simulink model "Citation"  (Simulink 10.1)
settings: Solver=ode5  StartTime=0.0  StopTime=inf  FixedStep=0.01  RelTol=1e-3  EnableMultiTasking=on
values from neighbouring files (symbols this model uses):
  S = 12.9900    (= 12.99)    [FTFC.m]
  Vw915 = 0    [initcit.m]
  winddir = 45*(pi/180)    (= 0.785398163397)    [initcit.m]
  x0 = []    [cessnac550_3d_sfnc.m]    (also in sfunxyz.m)
undefined symbols (not defined in the file or in its folder): chord, cv1, cv2, cv3, cv4, deltagmax1, deltagmax2, deltagmax3, deltagmax4, Deng, ealphag, ealphas, g0, hDME, hGS, kt1, kt2, kt3, lh, massinit, matbuaf, matdaf, matdam, matdbbf, matdeaf, matdgaf, matdqaf, matduaf, matdwaw, matedhr, mateif, matelhr, matemhr, matemv1, matemv2, matemve, matetam, mateuaf, matfaaf, matfaxl, matff, matibaf, matibmh, matipaf, matipmh, matiraf, matiuaf, matiwaf, matlaf, matlam, matleaf, matleam, matlgaf, matlqaf, matluaf, matmaaf, matmaam, matmaf, matmam, matmbbf ... (+74)
undefined symbols (not defined in the file): matibb
libraries: simulink x12, vrlib x1
(part 4 of 5)

== system Citation/Cessna Citation 500/Citation model DASMAT/AIRCRAFT MODEL/LANDING GEAR/Landing Gear model/Right Main Gear/Axes Transformation Heading attached vertical axis to body axis ==
  Fmu FS FV phi theta : Inport
  FX : Fcn  Expr=-cos(u[5])*u[1]+0*u[2]+sin(u[5])*u[3]
  FY : Fcn  Expr=-sin(u[5])*sin(u[4])*u[1]-cos(u[4])*u[2]-cos(u[5])*sin(u[4])*u[3]
  FZ : Fcn  Expr=-sin(u[5])*cos(u[4])*u[1]+sin(u[4])*u[2]-cos(u[5])*cos(u[4])*u[3]
  Mux1 : Mux  Inputs=3
  FX FY FZ : Outport
  wires:
  Fmu FS FV phi theta/1 -> FX/1, FY/1, FZ/1
  FX/1 -> Mux1/1
  FY/1 -> Mux1/2
  FZ/1 -> Mux1/3
  Mux1/1 -> FX FY FZ/1

== system Citation/Cessna Citation 500/Citation model DASMAT/AIRCRAFT MODEL/LANDING GEAR/Landing Gear model/Right Main Gear/Calculation of the Moments ==
  FX FY FZ : Inport
  L : Fcn  Expr=0*u[1]-zl2*u[2]+yl2*u[3]
  M : Fcn  Expr=zl2*u[1]+0*u[2]-xl2*u[3]
  Mux2 : Mux  Inputs=3
  N : Fcn  Expr=-yl2*u[1]+xl2*u[2]+0*u[3]
  L M N : Outport
  wires:
  L/1 -> Mux2/1
  M/1 -> Mux2/2
  N/1 -> Mux2/3
  FX FY FZ/1 -> M/1, L/1, N/1
  Mux2/1 -> L M N/1

== system Citation/Cessna Citation 500/Citation model DASMAT/AIRCRAFT MODEL/LANDING GEAR/Landing Gear model/Right Main Gear/FV Vertical Force ==
  In1 : Inport
  B : Fcn  Expr=(u[2]/kt2)-u[1]-deltagmax2
  C : Fcn  Expr=(deltagmax2/kt2)*(P2+u[2]-(kt2*u[1]))
  FD damping force : Fcn  Expr=cv2*u[1]
  FV : Fcn  Expr=kt2*(u[1]-u[2])
  FV No ground contact : Constant  Value=0
  Mux1 : Mux  Inputs=2
  Mux2 : Mux  Inputs=2
  Mux3 : Mux  Inputs=2
  No negative  Strut deflection : Saturate  UpperLimit=inf  LowerLimit=0
  Prevent Earth  from pulling a/c when FD>FV : Saturate  UpperLimit=inf  LowerLimit=0
  Strut deflection : Fcn  Expr=0.5*(-u[1]-sqrt(u[1]*u[1]+4*u[2]))
  Switch1 : Switch  SaturateOnIntegerOverflow=on  InputSameDT=on
  deltag : Fcn  Expr=zl2-u[10]-xl2*sin(u[8])+yl2*sin(u[7])
  deltagdot : Fcn  Expr=-u[13]-xl2*u[2]*cos(u[8])+yl2*u[1]*cos(u[7])
  Out1 : Outport
  wires:
  In1/1 -> deltag/1, deltagdot/1
  deltagdot/1 -> FD damping force/1
  Strut deflection/1 -> No negative  Strut deflection/1
  FD damping force/1 -> Mux1/2
  Mux1/1 -> B/1, C/1
  B/1 -> Mux2/1
  C/1 -> Mux2/2
  Mux2/1 -> Strut deflection/1
  Mux3/1 -> FV/1
  No negative  Strut deflection/1 -> Mux3/2
  deltag/1 -> Mux1/1, Mux3/1, Switch1/2
  FV/1 -> Prevent Earth  from pulling a/c when FD>FV/1
  FV No ground contact/1 -> Switch1/3
  Prevent Earth  from pulling a/c when FD>FV/1 -> Switch1/1
  Switch1/1 -> Out1/1

== system Citation/Cessna Citation 500/Citation model DASMAT/AIRCRAFT MODEL/LANDING GEAR/Landing Gear model/Tail Scraper/Axes Transformation Heading attached vertical axis to body axis ==
  Fmu FS FV phi theta : Inport
  FX : Fcn  Expr=-cos(u[5])*u[1]+0*u[2]+sin(u[5])*u[3]
  FY : Fcn  Expr=-sin(u[5])*sin(u[4])*u[1]-cos(u[4])*u[2]-cos(u[5])*sin(u[4])*u[3]
  FZ : Fcn  Expr=-sin(u[5])*cos(u[4])*u[1]+sin(u[4])*u[2]-cos(u[5])*cos(u[4])*u[3]
  Mux1 : Mux  Inputs=3
  FX FY FZ : Outport
  wires:
  Fmu FS FV phi theta/1 -> FX/1, FY/1, FZ/1
  FX/1 -> Mux1/1
  FY/1 -> Mux1/2
  FZ/1 -> Mux1/3
  Mux1/1 -> FX FY FZ/1

== system Citation/Cessna Citation 500/Citation model DASMAT/AIRCRAFT MODEL/LANDING GEAR/Landing Gear model/Tail Scraper/Calculation of the Moments ==
  FX FY FZ : Inport
  L : Fcn  Expr=0*u[1]-zl4*u[2]+yl4*u[3]
  M : Fcn  Expr=zl4*u[1]+0*u[2]-xl4*u[3]
  Mux2 : Mux  Inputs=3
  N : Fcn  Expr=-yl4*u[1]+xl4*u[2]+0*u[3]
  L M N : Outport
  wires:
  L/1 -> Mux2/1
  M/1 -> Mux2/2
  N/1 -> Mux2/3
  FX FY FZ/1 -> M/1, L/1, N/1
  Mux2/1 -> L M N/1

== system Citation/Cessna Citation 500/Citation model DASMAT/AIRCRAFT MODEL/LANDING GEAR/Landing Gear model/Tail Scraper/FV Vertical Force ==
  In1 : Inport
  FD damping force : Fcn  Expr=cv4*u[1]
  FV : Fcn  Expr=P4*u[1]+u[2]
  FV No ground contact : Constant  Value=0
  Max Strut Deflection : Saturate  UpperLimit=deltagmax4  LowerLimit=-inf
  Mux1 : Mux  Inputs=2
  Prevent Earth  from pulling a/c when FD>FV : Saturate  UpperLimit=inf  LowerLimit=0
  Scope6 : Scope
  Switch : Switch  SaturateOnIntegerOverflow=on  InputSameDT=on
  deltag : Fcn  Expr=zl4-u[10]-xl4*sin(u[8])+yl4*sin(u[7])
  deltagdot : Fcn  Expr=-u[13]-xl4*u[2]*cos(u[8])+yl4*u[1]*cos(u[7])
  Out1 : Outport
  wires:
  In1/1 -> deltag/1, deltagdot/1
  deltagdot/1 -> FD damping force/1
  deltag/1 -> Max Strut Deflection/1
  Max Strut Deflection/1 -> Scope6/1, Mux1/1, Switch/2
  Mux1/1 -> FV/1
  FD damping force/1 -> Mux1/2
  FV/1 -> Prevent Earth  from pulling a/c when FD>FV/1
  Prevent Earth  from pulling a/c when FD>FV/1 -> Switch/1
  FV No ground contact/1 -> Switch/3
  Switch/1 -> Out1/1

== system Citation/Cessna Citation 500/Citation model DASMAT/AIRCRAFT MODEL/WIND/TURBULENCE/Logarithmic Wind model/Logarithmic Wind model/Vwind915 ==
  Constant : Constant  Value=0
  Parameter : Integrator  InitialCondition=Vw915
  Out1 : Outport
  wires:
  Constant/1 -> Parameter/1
  Parameter/1 -> Out1/1

== system Citation/Cessna Citation 500/Citation model DASMAT/AIRCRAFT MODEL/WIND/TURBULENCE/Logarithmic Wind model/Logarithmic Wind model/Windddirection ==
  Constant : Constant  Value=0
  Parameter : Integrator  InitialCondition=winddir
  Out1 : Outport
  wires:
  Constant/1 -> Parameter/1
  Parameter/1 -> Out1/1

== system Citation/Cessna Citation 500/Citation model DASMAT/AIRCRAFT MODEL/AFM/Aeromod/SubSystem/model/CDCAL ==
  in_1 : Inport
  Abs : Abs  SaturateOnIntegerOverflow=on
  Abs1 : Abs  SaturateOnIntegerOverflow=on
  CD : Sum  Inputs=++++++++  InputSameDT=on  SaturateOnIntegerOverflow=on  OutDataTypeStr=Inherit: Same as first input
  CDAF : Lookup2D  RowIndex=matdaf(2:23,1)  ColumnIndex=matdaf(1,2:23)  Table=matdaf(2:23,2:23)  SaturateOnIntegerOverflow=on  InputSameDT=on
  CDAM : Lookup2D  RowIndex=matdam(2:23,1)  ColumnIndex=matdam(1,2:23)  Table=matdam(2:23,2:23)  SaturateOnIntegerOverflow=on  InputSameDT=on
  CDBAS : Sum  InputSameDT=on  SaturateOnIntegerOverflow=on  OutDataTypeStr=Inherit: Same as first input
  CDBBF : Lookup2D  RowIndex=matdbbf(2:18,1)  ColumnIndex=matdbbf(1,2:18)  Table=matdbbf(2:18,2:18)  SaturateOnIntegerOverflow=on  InputSameDT=on
  CDDE : Product  InputSameDT=on  SaturateOnIntegerOverflow=on  OutDataTypeStr=Inherit: Same as first input
  CDEAF : Lookup2D  RowIndex=matdeaf(2:23,1)  ColumnIndex=matdeaf(1,2:23)  Table=matdeaf(2:23,2:23)  SaturateOnIntegerOverflow=on  InputSameDT=on
  CDGAF : Lookup2D  RowIndex=matdgaf(2:4,1)  ColumnIndex=matdgaf(1,2:4)  Table=matdgaf(2:4,2:4)  SaturateOnIntegerOverflow=on  InputSameDT=on
  CDGE : Product  InputSameDT=on  SaturateOnIntegerOverflow=on  OutDataTypeStr=Inherit: Same as first input
  CDQ : Product  InputSameDT=on  SaturateOnIntegerOverflow=on  OutDataTypeStr=Inherit: Same as first input
  CDQAF : Lookup2D  RowIndex=matdqaf(2:23,1)  ColumnIndex=matdqaf(1,2:23)  Table=matdqaf(2:23,2:23)  SaturateOnIntegerOverflow=on  InputSameDT=on
  CDR : Product  Inputs=3  InputSameDT=on  SaturateOnIntegerOverflow=on  OutDataTypeStr=Inherit: Same as first input
  CDRUAF : Lookup2D  RowIndex=matruaf(2:3,1)  ColumnIndex=matruaf(1,2:3)  Table=matruaf(2:3,2:3)  SaturateOnIntegerOverflow=on  InputSameDT=on
  CDUAF : Lookup2D  RowIndex=matduaf(2:23,1)  ColumnIndex=matduaf(1,2:23)  Table=matduaf(2:23,2:23)  SaturateOnIntegerOverflow=on  InputSameDT=on
  CDUC : Product  InputSameDT=on  SaturateOnIntegerOverflow=on  OutDataTypeStr=Inherit: Same as first input
  CDWAW : Lookup2D  RowIndex=matdwaw(2:7,1)  ColumnIndex=matdwaw(1,2:7)  Table=matdwaw(2:7,2:7)  SaturateOnIntegerOverflow=on  InputSameDT=on
  Demux : Demux  Outputs=[1 1 1 1 1 1 1 1 1 1 1 1 1 1 1 1 1 1]
      settings: DisplayOption=none
  KBASD : Subsystem
  KGEDHR : Lookup  InputValues=matedhr(1,:)  Table=matedhr(2,:)  SaturateOnIntegerOverflow=on
  KUUT : Lookup  InputValues=matuut(1,:)  Table=matuut(2,:)  SaturateOnIntegerOverflow=on
  Prod : Product  InputSameDT=on  SaturateOnIntegerOverflow=on  OutDataTypeStr=Inherit: Same as first input
  Terminator_{1..7} (7 alike) : Terminator
  out_1 : Outport
  wires:
  Demux/16 -> Terminator_7/1
  Demux/13 -> Terminator_6/1
  Demux/12 -> Terminator_5/1
  Demux/11 -> Terminator_4/1
  Demux/6 -> Terminator_3/1
  Demux/3 -> Terminator_2/1
  Demux/1 -> Terminator_1/1
  Demux/7 -> KBASD/1(hcg), KGEDHR/1
  Demux/18 -> KBASD/3(VEAS)
  Demux/2 -> CDQ/1
  Demux/5 -> Abs1/1
  Demux/8 -> CDDE/1
  Demux/9 -> Abs/1
  Demux/15 -> KUUT/1
  Demux/17 -> CDAM/1
  KUUT/1 -> CDUC/2
  CDGAF/1 -> CDGE/1
  CDR/1 -> CD/6
  CDQ/1 -> CD/5
  CDWAW/1 -> CD/3
  CDDE/1 -> CD/2
  CDRUAF/1 -> CDR/3
  CDQAF/1 -> CDQ/2
  CDEAF/1 -> CDDE/2
  Abs/1 -> CDWAW/1
  Abs1/1 -> CDBBF/2
  CD/1 -> out_1/1
  Demux/10 -> CDR/1, CDR/2
  Demux/14 -> CDAF/1, CDRUAF/1, CDUAF/1, CDGAF/1, CDQAF/1, CDBBF/1, CDEAF/1, KBASD/2(deltaf)
  KGEDHR/1 -> CDGE/2
  Demux/4 -> CDRUAF/2, CDUAF/2, CDGAF/2, CDQAF/2, CDWAW/2, CDEAF/2, CDAF/2, CDAM/2
  CDAF/1 -> Prod/1
  KBASD/1(KBASD) -> Prod/2
  CDUAF/1 -> CDUC/1
  CDUC/1 -> CD/7
  CDGE/1 -> CD/8
  CDBBF/1 -> CD/4
  Prod/1 -> CDBAS/2
  CDAM/1 -> CDBAS/1
  CDBAS/1 -> CD/1
  in_1/1 -> Demux/1

== system Citation/Cessna Citation 500/Citation model DASMAT/AIRCRAFT MODEL/AFM/Aeromod/SubSystem/model/CLCAL ==
  in_1 : Inport
  CL : Sum  Inputs=+++++  InputSameDT=on  SaturateOnIntegerOverflow=on  OutDataTypeStr=Inherit: Same as first input
  CLADOT : Product  InputSameDT=on  SaturateOnIntegerOverflow=on  OutDataTypeStr=Inherit: Same as first input
  CLAF : Lookup2D  RowIndex=matlaf(2:23,1)  ColumnIndex=matlaf(1,2:23)  Table=matlaf(2:23,2:23)  SaturateOnIntegerOverflow=on  InputSameDT=on
  CLAM : Lookup2D  RowIndex=matlam(2:23,1)  ColumnIndex=matlam(1,2:23)  Table=matlam(2:23,2:23)  SaturateOnIntegerOverflow=on  InputSameDT=on
  CLBAS : Sum  InputSameDT=on  SaturateOnIntegerOverflow=on  OutDataTypeStr=Inherit: Same as first input
  CLDE : Product  InputSameDT=on  SaturateOnIntegerOverflow=on  OutDataTypeStr=Inherit: Same as first input
  CLEAF : Lookup2D  RowIndex=matleaf(2:23,1)  ColumnIndex=matleaf(1,2:23)  Table=matleaf(2:23,2:23)  SaturateOnIntegerOverflow=on  InputSameDT=on
  CLEAM : Lookup2D  RowIndex=matleam(2:3,1)  ColumnIndex=matleam(1,2:3)  Table=matleam(2:3,2:3)  SaturateOnIntegerOverflow=on  InputSameDT=on
  CLFAAF : Lookup2D  RowIndex=matfaaf(2:23,1)  ColumnIndex=matfaaf(1,2:23)  Table=matfaaf(2:23,2:23)  SaturateOnIntegerOverflow=on  InputSameDT=on
  CLGAF : Lookup2D  RowIndex=matlgaf(2:4,1)  ColumnIndex=matlgaf(1,2:4)  Table=matlgaf(2:4,2:4)  SaturateOnIntegerOverflow=on  InputSameDT=on
  CLGE : Product  InputSameDT=on  SaturateOnIntegerOverflow=on  OutDataTypeStr=Inherit: Same as first input
  CLGEAF : Subsystem
  CLQ : Product  Inputs=3  InputSameDT=on  SaturateOnIntegerOverflow=on  OutDataTypeStr=Inherit: Same as first input
  CLQAF : Lookup2D  RowIndex=matlqaf(2:23,1)  ColumnIndex=matlqaf(1,2:23)  Table=matlqaf(2:23,2:23)  SaturateOnIntegerOverflow=on  InputSameDT=on
  CLQUAF : Lookup2D  RowIndex=matqlaf(2:3,1)  ColumnIndex=matqlaf(1,2:3)  Table=matqlaf(2:3,2:3)  SaturateOnIntegerOverflow=on  InputSameDT=on
  CLUAF : Lookup2D  RowIndex=matluaf(2:23,1)  ColumnIndex=matluaf(1,2:23)  Table=matluaf(2:23,2:23)  SaturateOnIntegerOverflow=on  InputSameDT=on
  CLUC : Product  InputSameDT=on  SaturateOnIntegerOverflow=on  OutDataTypeStr=Inherit: Same as first input
  Demux : Demux  Outputs=[1 1 1 1 1 1 1 1 1 1 1 1 1 1 1 1 1 1]
      settings: DisplayOption=none
  Gain : Gain  Gain=0.01  SaturateOnIntegerOverflow=on  OutDataTypeStr=Inherit: Same as input  ParamDataTypeStr=Inherit: Same as input
  KFAXL : Lookup  InputValues=matfaxl(1,:)  Table=matfaxl(2,:)  SaturateOnIntegerOverflow=on
  KGELHR : Lookup  InputValues=matelhr(1,:)  Table=matelhr(2,:)  SaturateOnIntegerOverflow=on
  KQXL : Lookup  InputValues=matqxl(1,:)  Table=matqxl(2,:)  SaturateOnIntegerOverflow=on
  KUUT : Lookup  InputValues=matuut(1,:)  Table=matuut(2,:)  SaturateOnIntegerOverflow=on
  Prod : Product  InputSameDT=on  SaturateOnIntegerOverflow=on  OutDataTypeStr=Inherit: Same as first input
  SP0 : Subsystem
  Sum : Sum  InputSameDT=on  SaturateOnIntegerOverflow=on  OutDataTypeStr=Inherit: Same as first input
  Sum1 : Sum  Inputs=2  InputSameDT=on  SaturateOnIntegerOverflow=on  OutDataTypeStr=Inherit: Same as first input
  Sum2 : Sum  Inputs=2  InputSameDT=on  SaturateOnIntegerOverflow=on  OutDataTypeStr=Inherit: Same as first input
  Terminator_{1..10} (10 alike) : Terminator
  out_1 : Outport
  out_2 : Outport  Port=2
  wires:
  Demux/18 -> Terminator_10/1
  Demux/13 -> Terminator_9/1
  Demux/12 -> Terminator_8/1
  Demux/11 -> Terminator_7/1
  Demux/10 -> Terminator_6/1
  Demux/9 -> Terminator_5/1
  Demux/6 -> Terminator_4/1
  Demux/5 -> Terminator_3/1
  Demux/3 -> Terminator_2/1
  Demux/1 -> Terminator_1/1
  CLADOT/1 -> out_2/1
  CLFAAF/1 -> CLADOT/1
  CLAF/1 -> CLBAS/2
  CLDE/1 -> CL/2
  Sum/1 -> CLDE/1
  SP0/1(SP0) -> CLDE/2
  CLQ/1 -> CL/3
  CL/1 -> out_1/1
  CLQUAF/1 -> Prod/2
  Sum1/1 -> CLUC/1
  CLQAF/1 -> CLQ/2
  Prod/1 -> Sum1/2
  CLUAF/1 -> Sum1/1
  CLGAF/1 -> Sum2/1
  KGELHR/1 -> CLGE/2
  KFAXL/1 -> Gain/1
  Gain/1 -> CLADOT/2
  Demux/14 -> CLAF/1, CLEAF/1, CLQAF/1, CLUAF/1, CLQUAF/1, CLGAF/1, CLGEAF/2(deltaf), CLFAAF/1
  CLEAF/1 -> Sum/2
  CLEAM/1 -> Sum/1
  CLUC/1 -> CL/4
  CLGE/1 -> CL/5
  CLGEAF/1(CLGEAF) -> Sum2/2
  in_1/1 -> Demux/1
  Demux/17 -> CLAM/1, CLEAM/1
  Demux/4 -> CLAM/2, CLAF/2, CLEAM/2, CLEAF/2, CLQAF/2, CLUAF/2, CLQUAF/2, CLGAF/2, CLGEAF/1(alpha), CLFAAF/2
  CLBAS/1 -> CL/1
  Demux/2 -> CLQ/1, Prod/1
  KQXL/1 -> CLQ/3
  KUUT/1 -> CLUC/2
  CLAM/1 -> CLBAS/1
  Demux/15 -> KQXL/1, KUUT/1
  Sum2/1 -> CLGE/1
  Demux/16 -> KFAXL/1
  Demux/8 -> SP0/1(deltae)
  Demux/7 -> KGELHR/1

== system Citation/Cessna Citation 500/Citation model DASMAT/AIRCRAFT MODEL/AFM/Aeromod/SubSystem/model/CLLCAL ==
  in_1 : Inport
  Abs : Abs  SaturateOnIntegerOverflow=on
  CIBAB : Subsystem  mask(3-D Table Lookup){xindex=matibb(2:5,1), yindex=matibb(1,2:4), zindex=matibb(1,5:7), table=matibb(2:5,2:10)}
      mask prompts: xindex "X Index"; yindex "Y Index"; zindex "Z Index"
      mask help:
      | Three Dimensional Table Lookup
      | The first, second and third input corresponds to the X,Y and Z Index
      mask Help: This block returns a linearly interpolated intersection from the table using the X index (which corresponds to the rows of the table), the Y index (which corresponds to the columns of the table) and the Z index.  Extrapolation is used.
      mask Display: plot(-10,-10,110,110,[90,50,10],[90,40,30],[90,50,10],[50,26,20],[90,50,10],[22,13,10])
  CIBAF : Lookup2D  RowIndex=matibaf(2:4,1)  ColumnIndex=matibaf(1,2:4)  Table=matibaf(2:4,2:4)  SaturateOnIntegerOverflow=on  InputSameDT=on
  CIBMH : Lookup2D  RowIndex=matibmh(2:10,1)  ColumnIndex=matibmh(1,2:10)  Table=matibmh(2:10,2:10)  SaturateOnIntegerOverflow=on  InputSameDT=on
  CIPAF : Lookup2D  RowIndex=matipaf(2:3,1)  ColumnIndex=matipaf(1,2:3)  Table=matipaf(2:3,2:3)  SaturateOnIntegerOverflow=on  InputSameDT=on
  CIPMH : Lookup2D  RowIndex=matipmh(2:10,1)  ColumnIndex=matipmh(1,2:10)  Table=matipmh(2:10,2:10)  SaturateOnIntegerOverflow=on  InputSameDT=on
  CIRAF : Lookup2D  RowIndex=matiraf(2:4,1)  ColumnIndex=matiraf(1,2:4)  Table=matiraf(2:4,2:4)  SaturateOnIntegerOverflow=on  InputSameDT=on
  CIRUAF : Lookup2D  RowIndex=matiuaf(2:3,1)  ColumnIndex=matiuaf(1,2:3)  Table=matiuaf(2:3,2:3)  SaturateOnIntegerOverflow=on  InputSameDT=on
  CIRUMH : Lookup2D  RowIndex=matrumh(2:10,1)  ColumnIndex=matrumh(1,2:10)  Table=matrumh(2:10,2:10)  SaturateOnIntegerOverflow=on  InputSameDT=on
  CIWAF : Lookup2D  RowIndex=matiwaf(2:3,1)  ColumnIndex=matiwaf(1,2:3)  Table=matiwaf(2:3,2:3)  SaturateOnIntegerOverflow=on  InputSameDT=on
  CIWTAM : Lookup2D  RowIndex=matwtam(2:3,1)  ColumnIndex=matwtam(1,2:3)  Table=matwtam(2:3,2:3)  SaturateOnIntegerOverflow=on  InputSameDT=on
  CLL : Sum  Inputs=+++++++  InputSameDT=on  SaturateOnIntegerOverflow=on  OutDataTypeStr=Inherit: Same as first input
  CLLB : Product  InputSameDT=on  SaturateOnIntegerOverflow=on  OutDataTypeStr=Inherit: Same as first input
  CLLDA : Product  InputSameDT=on  SaturateOnIntegerOverflow=on  OutDataTypeStr=Inherit: Same as first input
  CLLDR : Product  InputSameDT=on  SaturateOnIntegerOverflow=on  OutDataTypeStr=Inherit: Same as first input
  CLLGE : Product  Inputs=3  InputSameDT=on  SaturateOnIntegerOverflow=on  OutDataTypeStr=Inherit: Same as first input
  CLLGUST : Mux  Inputs=8
  CLLP : Product  InputSameDT=on  SaturateOnIntegerOverflow=on  OutDataTypeStr=Inherit: Same as first input
  CLLR : Product  InputSameDT=on  SaturateOnIntegerOverflow=on  OutDataTypeStr=Inherit: Same as first input
  CLLTRIM : Product  InputSameDT=on  SaturateOnIntegerOverflow=on  OutDataTypeStr=Inherit: Same as first input
  Demux1 : Demux  Outputs=[1 1 1 1 1 1 1 1 1 1 1 1 1 1 1 1 1 1]
      settings: DisplayOption=none
  LFACT : Subsystem
  LROLL : Lookup  InputValues=mateif(1,:)  Table=mateif(2,:)  SaturateOnIntegerOverflow=on
  Sum : Sum  Inputs=+++  InputSameDT=on  SaturateOnIntegerOverflow=on  OutDataTypeStr=Inherit: Same as first input
  Sum1 : Sum  InputSameDT=on  SaturateOnIntegerOverflow=on  OutDataTypeStr=Inherit: Same as first input
  Sum2 : Sum  InputSameDT=on  SaturateOnIntegerOverflow=on  OutDataTypeStr=Inherit: Same as first input
  Terminator_{1..7} (7 alike) : Terminator
  "neg " : Gain  Gain=-1  SaturateOnIntegerOverflow=on  OutDataTypeStr=Inherit: Same as input  ParamDataTypeStr=Inherit: Same as input
  zero : Constant  Value=0
  out_1 : Outport
  out_2 : Outport  Port=2
  wires:
  Demux1/18 -> Terminator_7/1
  Demux1/16 -> Terminator_6/1
  Demux1/15 -> Terminator_5/1
  Demux1/13 -> Terminator_4/1
  Demux1/11 -> Terminator_3/1
  Demux1/8 -> Terminator_2/1
  Demux1/2 -> Terminator_1/1
  Sum/1 -> CLLGUST/3, CLLB/2
  LFACT/1(LFACT) -> CLLGE/3
  LROLL/1 -> CLLGE/2
  CLL/1 -> out_1/1
  CLLB/1 -> CLL/1
  CIWTAM/1 -> CLLTRIM/2
  CIWAF/1 -> CLLDA/2
  Sum1/1 -> CLLDR/2
  CIRUMH/1 -> Sum1/2
  Abs/1 -> CIBAB/1(x0)
  CIRUAF/1 -> Sum1/1
  CIBAF/1 -> Sum/1
  CIPAF/1 -> Sum2/1
  CIPMH/1 -> Sum2/2
  Demux1/14 -> CIBAF/1, CIRUAF/1, CIRAF/1, LROLL/1, CIPAF/1, CIWAF/1, CIBAB/3(z0)
  Demux1/5 -> CLLB/1, Abs/1, CLLGE/1
  Demux1/4 -> CIWAF/2, CIRUAF/2, CIPAF/2, CIRAF/2, CIWTAM/2, CIBAB/2(y0), CIBAF/2
  zero/1 -> CLLGUST/2, CLLGUST/5, CLLGUST/6, CLLGUST/4, CLLGUST/1
  CLLGUST/1 -> out_2/1
  CIRAF/1 -> "neg "/1, CLLR/2
  Sum2/1 -> CLLGUST/8, CLLP/2
  "neg "/1 -> CLLGUST/7
  in_1/1 -> Demux1/1
  CLLGE/1 -> CLL/7
  CLLR/1 -> CLL/6
  CLLTRIM/1 -> CLL/4
  CLLDA/1 -> CLL/2
  Demux1/12 -> CLLTRIM/1
  Demux1/10 -> CLLDR/1
  Demux1/9 -> CLLDA/1
  Demux1/1 -> CLLP/1
  Demux1/3 -> CLLR/1
  CIBMH/1 -> Sum/2
  CIBAB/1(out_1) -> Sum/3
  Demux1/17 -> CIRUMH/2, CIWTAM/1, CIPMH/2, CIBMH/2
  Demux1/6 -> CIRUMH/1, CIPMH/1, CIBMH/1
  Demux1/7 -> LFACT/1(hcg)
  CLLP/1 -> CLL/5
  CLLDR/1 -> CLL/3

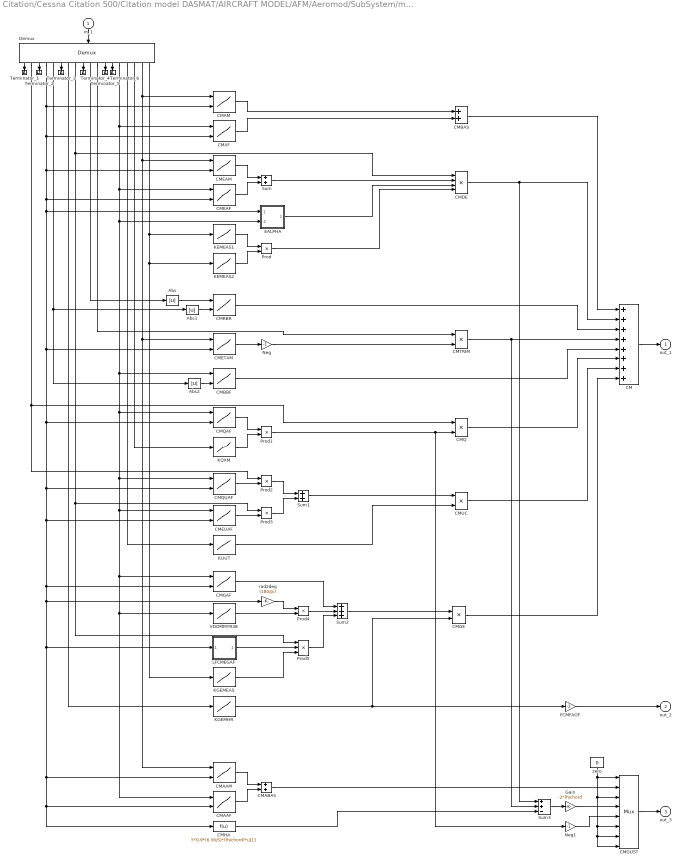
== system Citation/Cessna Citation 500/Citation model DASMAT/AIRCRAFT MODEL/AFM/Aeromod/SubSystem/model/CMCAL ==
  in_1 : Inport
  Abs : Abs  SaturateOnIntegerOverflow=on
  Abs1 : Abs  SaturateOnIntegerOverflow=on
  Abs2 : Abs  SaturateOnIntegerOverflow=on
  CM : Sum  Inputs=++++++++  InputSameDT=on  SaturateOnIntegerOverflow=on  OutDataTypeStr=Inherit: Same as first input
  CMAAF : Lookup2D  RowIndex=matmaaf(2:22,1)  ColumnIndex=matmaaf(1,2:22)  Table=matmaaf(2:22,2:22)  SaturateOnIntegerOverflow=on  InputSameDT=on
  CMAAM : Lookup2D  RowIndex=matmaam(2:22,1)  ColumnIndex=matmaam(1,2:22)  Table=matmaam(2:22,2:22)  SaturateOnIntegerOverflow=on  InputSameDT=on
  CMABAS : Sum  InputSameDT=on  SaturateOnIntegerOverflow=on  OutDataTypeStr=Inherit: Same as first input
  CMAF : Lookup2D  RowIndex=matmaf(2:23,1)  ColumnIndex=matmaf(1,2:23)  Table=matmaf(2:23,2:23)  SaturateOnIntegerOverflow=on  InputSameDT=on
  "CMAM " : Lookup2D  RowIndex=matmam(2:23,1)  ColumnIndex=matmam(1,2:23)  Table=matmam(2:23,2:23)  SaturateOnIntegerOverflow=on  InputSameDT=on
  CMBAS : Sum  InputSameDT=on  SaturateOnIntegerOverflow=on  OutDataTypeStr=Inherit: Same as first input
  CMBBF : Lookup2D  RowIndex=matmbbf(2:18,1)  ColumnIndex=matmbbf(1,2:18)  Table=matmbbf(2:18,2:18)  SaturateOnIntegerOverflow=on  InputSameDT=on
  CMDE : Product  Inputs=4  InputSameDT=on  SaturateOnIntegerOverflow=on  OutDataTypeStr=Inherit: Same as first input
  CMEAF : Lookup2D  RowIndex=matmeaf(2:23,1)  ColumnIndex=matmeaf(1,2:23)  Table=matmeaf(2:23,2:23)  SaturateOnIntegerOverflow=on  InputSameDT=on
  CMEAM : Lookup2D  RowIndex=matmeam(2:23,1)  ColumnIndex=matmeam(1,2:23)  Table=matmeam(2:23,2:23)  SaturateOnIntegerOverflow=on  InputSameDT=on
  CMETAM : Lookup2D  RowIndex=matetam(2:3,1)  ColumnIndex=matetam(1,2:3)  Table=matetam(2:3,2:3)  SaturateOnIntegerOverflow=on  InputSameDT=on
  CMEUAF : Lookup2D  RowIndex=mateuaf(2:23,1)  ColumnIndex=mateuaf(1,2:23)  Table=mateuaf(2:23,2:23)  SaturateOnIntegerOverflow=on  InputSameDT=on
  CMGAF : Lookup2D  RowIndex=matmgaf(2:4,1)  ColumnIndex=matmgaf(1,2:4)  Table=matmgaf(2:4,2:4)  SaturateOnIntegerOverflow=on  InputSameDT=on
  CMGE : Product  InputSameDT=on  SaturateOnIntegerOverflow=on  OutDataTypeStr=Inherit: Same as first input
  CMGUST : Mux  Inputs=8
  CMHA : Fcn  Expr=5*0.9*(6.56/S)*(lh/chord)*u[1]
  CMQ : Product  InputSameDT=on  SaturateOnIntegerOverflow=on  OutDataTypeStr=Inherit: Same as first input
  CMQAF : Lookup2D  RowIndex=matmqaf(2:23,1)  ColumnIndex=matmqaf(1,2:23)  Table=matmqaf(2:23,2:23)  SaturateOnIntegerOverflow=on  InputSameDT=on
  CMQUAF : Lookup2D  RowIndex=matquaf(2:23,1)  ColumnIndex=matquaf(1,2:23)  Table=matquaf(2:23,2:23)  SaturateOnIntegerOverflow=on  InputSameDT=on
  CMRBR : Lookup2D  RowIndex=matmrbr(2:3,1)  ColumnIndex=matmrbr(1,2:3)  Table=matmrbr(2:3,2:3)  SaturateOnIntegerOverflow=on  InputSameDT=on
  CMTRIM : Product  InputSameDT=on  SaturateOnIntegerOverflow=on  OutDataTypeStr=Inherit: Same as first input
  CMUC : Product  InputSameDT=on  SaturateOnIntegerOverflow=on  OutDataTypeStr=Inherit: Same as first input
  Demux : Demux  Outputs=[1 1 1 1 1 1 1 1 1 1 1 1 1 1 1 1 1 1]
      settings: DisplayOption=none
  EALPHA : Subsystem
  FCMFAGF : Gain  Gain=-2  SaturateOnIntegerOverflow=on  OutDataTypeStr=Inherit: Same as input  ParamDataTypeStr=Inherit: Same as input
  Gain : Gain  Gain=-2*lh/chord  SaturateOnIntegerOverflow=on  OutDataTypeStr=Inherit: Same as input  ParamDataTypeStr=Inherit: Same as input
  KEMEAS1 : Lookup  InputValues=matemv1(1,:)  Table=matemv1(2,:)  SaturateOnIntegerOverflow=on
  KEMEAS2 : Lookup  InputValues=matemv2(1,:)  Table=matemv2(2,:)  SaturateOnIntegerOverflow=on
  KGEMEAS : Lookup  InputValues=matemve(1,:)  Table=matemve(2,:)  SaturateOnIntegerOverflow=on
  KGEMHR : Lookup  InputValues=matemhr(1,:)  Table=matemhr(2,:)  SaturateOnIntegerOverflow=on
  KQXM : Lookup  InputValues=matqxm(1,:)  Table=matqxm(2,:)  SaturateOnIntegerOverflow=on
  KUUT : Lookup  InputValues=matuut(1,:)  Table=matuut(2,:)  SaturateOnIntegerOverflow=on
  LFCMEGAF : Subsystem
  "Neg " : Gain  Gain=-1  SaturateOnIntegerOverflow=on  OutDataTypeStr=Inherit: Same as input  ParamDataTypeStr=Inherit: Same as input
  Neg1 : Gain  Gain=-1  SaturateOnIntegerOverflow=on  OutDataTypeStr=Inherit: Same as input  ParamDataTypeStr=Inherit: Same as input
  Prod{,1..4} (5 alike) : Product  InputSameDT=on  SaturateOnIntegerOverflow=on  OutDataTypeStr=Inherit: Same as first input
  Prod5 : Product  Inputs=3  InputSameDT=on  SaturateOnIntegerOverflow=on  OutDataTypeStr=Inherit: Same as first input
  Sum : Sum  InputSameDT=on  SaturateOnIntegerOverflow=on  OutDataTypeStr=Inherit: Same as first input
  Sum1 : Sum  InputSameDT=on  SaturateOnIntegerOverflow=on  OutDataTypeStr=Inherit: Same as first input
  Sum2 : Sum  Inputs=+++  InputSameDT=on  SaturateOnIntegerOverflow=on  OutDataTypeStr=Inherit: Same as first input
  Sum3 : Sum  Inputs=++-  InputSameDT=on  SaturateOnIntegerOverflow=on  OutDataTypeStr=Inherit: Same as first input
  Terminator_{1..6} (6 alike) : Terminator
  VDOMMYR38 : Lookup  InputValues=vdommyr38(1,:)  Table=vdommyr38(2,:)  SaturateOnIntegerOverflow=on
  rad2deg : Gain  Gain=(180/pi)  SaturateOnIntegerOverflow=on  OutDataTypeStr=Inherit: Same as input  ParamDataTypeStr=Inherit: Same as input
  zero : Constant  Value=0
  out_1 : Outport
  out_2 : Outport  Port=2
  "out_3 " : Outport  Port=3
  wires:
  Demux/13 -> Terminator_6/1
  Demux/12 -> Terminator_5/1
  Demux/9 -> Terminator_4/1
  Demux/6 -> Terminator_3/1
  Demux/3 -> Terminator_2/1
  Demux/1 -> Terminator_1/1
  Neg1/1 -> CMGUST/5
  CMABAS/1 -> CMGUST/2
  CMHA/1 -> Sum3/3
  CMGAF/1 -> Sum2/1
  Prod4/1 -> Sum2/2
  VDOMMYR38/1 -> Prod4/2
  CMQUAF/1 -> Prod2/2
  EALPHA/1(EALPHA) -> CMDE/3
  CMBAS/1 -> CM/1
  "CMAM "/1 -> CMBAS/1
  Abs/1 -> CMRBR/1
  Abs2/1 -> CMBBF/2
  KUUT/1 -> CMUC/2
  Sum1/1 -> CMUC/1
  Demux/14 -> CMAF/1, CMEAF/1, EALPHA/2(deltaf), CMQAF/1, CMQUAF/1, CMGAF/1, VDOMMYR38/1, CMAAF/1, CMEUAF/1, CMBBF/1
  Sum/1 -> CMDE/2
  Demux/8 -> CMDE/1, Prod3/1, Prod5/1
  Prod/1 -> CMDE/4
  Demux/18 -> KEMEAS1/1, KEMEAS2/1, KGEMEAS/1
  Demux/2 -> CMQ/1, Prod2/1
  CMETAM/1 -> "Neg "/1
  "Neg "/1 -> CMTRIM/2
  CMEUAF/1 -> Prod3/2
  Sum3/1 -> Gain/1
  Prod2/1 -> Sum1/1
  Sum2/1 -> CMGE/1
  Demux/4 -> "CMAM "/2, CMEAM/2, CMEAF/2, EALPHA/1(alpha), CMQAF/2, CMQUAF/2, CMEUAF/2, CMGAF/2, rad2deg/1, CMAAF/2, CMHA/1, CMAAM/2, LFCMEGAF/1(alpha), CMETAM/2, CMAF/2
  Demux/17 -> "CMAM "/1, CMEAM/1, CMETAM/1, CMAAM/1
  CMUC/1 -> CM/7
  CM/1 -> out_1/1
  CMGE/1 -> CM/8
  Prod1/1 -> Neg1/1, CMQ/2
  FCMFAGF/1 -> out_2/1
  CMGUST/1 -> "out_3 "/1
  Gain/1 -> CMGUST/4
  zero/1 -> CMGUST/6, CMGUST/7, CMGUST/8, CMGUST/3, CMGUST/1
  in_1/1 -> Demux/1
  Abs1/1 -> CMRBR/2
  Demux/5 -> Abs1/1, Abs2/1
  CMQAF/1 -> Prod1/1
  Prod3/1 -> Sum1/2
  CMRBR/1 -> CM/3
  CMQ/1 -> CM/6
  CMBBF/1 -> CM/5
  CMTRIM/1 -> Sum3/2, CM/4
  CMDE/1 -> Sum3/1, CM/2
  CMAF/1 -> CMBAS/2
  CMEAM/1 -> Sum/1
  CMEAF/1 -> Sum/2
  KQXM/1 -> Prod1/2
  CMAAM/1 -> CMABAS/1
  CMAAF/1 -> CMABAS/2
  Demux/16 -> KQXM/1
  Demux/15 -> KUUT/1
  Demux/11 -> CMTRIM/1
  Demux/10 -> Abs/1
  Demux/7 -> KGEMHR/1
  KEMEAS1/1 -> Prod/1
  KEMEAS2/1 -> Prod/2
  LFCMEGAF/1(LFCMEGAF) -> Prod5/2
  KGEMEAS/1 -> Prod5/3
  rad2deg/1 -> Prod4/1
  Prod5/1 -> Sum2/3
  KGEMHR/1 -> FCMFAGF/1, CMGE/2

== system Citation/Cessna Citation 500/Citation model DASMAT/AIRCRAFT MODEL/AFM/Aeromod/SubSystem/model/CNCAL ==
  in_1 : Inport
  Abs : Abs  SaturateOnIntegerOverflow=on
  CN : Sum  Inputs=++++++  InputSameDT=on  SaturateOnIntegerOverflow=on  OutDataTypeStr=Inherit: Same as first input
  CNB : Product  InputSameDT=on  SaturateOnIntegerOverflow=on  OutDataTypeStr=Inherit: Same as first input
  CNBAB : Lookup2D  RowIndex=matnbab(2:5,1)  ColumnIndex=matnbab(1,2:5)  Table=matnbab(2:5,2:5)  SaturateOnIntegerOverflow=on  InputSameDT=on
  CNBAF : Lookup2D  RowIndex=matnbaf(2:3,1)  ColumnIndex=matnbaf(1,2:3)  Table=matnbaf(2:3,2:3)  SaturateOnIntegerOverflow=on  InputSameDT=on
  CNBMH : Lookup2D  RowIndex=matnbmh(2:10,1)  ColumnIndex=matnbmh(1,2:10)  Table=matnbmh(2:10,2:10)  SaturateOnIntegerOverflow=on  InputSameDT=on
  CNDA : Product  InputSameDT=on  SaturateOnIntegerOverflow=on  OutDataTypeStr=Inherit: Same as first input
  CNDR : Product  InputSameDT=on  SaturateOnIntegerOverflow=on  OutDataTypeStr=Inherit: Same as first input
  CNGUST : Mux  Inputs=8
  CNP : Product  InputSameDT=on  SaturateOnIntegerOverflow=on  OutDataTypeStr=Inherit: Same as first input
  CNPAF : Lookup2D  RowIndex=matnpaf(2:4,1)  ColumnIndex=matnpaf(1,2:4)  Table=matnpaf(2:4,2:4)  SaturateOnIntegerOverflow=on  InputSameDT=on
  CNPMH : Lookup2D  RowIndex=matnpmh(2:10,1)  ColumnIndex=matnpmh(1,2:10)  Table=matnpmh(2:10,2:10)  SaturateOnIntegerOverflow=on  InputSameDT=on
  CNR : Product  InputSameDT=on  SaturateOnIntegerOverflow=on  OutDataTypeStr=Inherit: Same as first input
  CNRAF : Lookup2D  RowIndex=matnraf(2:3,1)  ColumnIndex=matnraf(1,2:3)  Table=matnraf(2:3,2:3)  SaturateOnIntegerOverflow=on  InputSameDT=on
  CNRTAM : Lookup2D  RowIndex=matrtam(2:3,1)  ColumnIndex=matrtam(1,2:3)  Table=matrtam(2:3,2:3)  SaturateOnIntegerOverflow=on  InputSameDT=on
  CNRUAF : Lookup2D  RowIndex=matnuaf(2:3,1)  ColumnIndex=matnuaf(1,2:3)  Table=matnuaf(2:3,2:3)  SaturateOnIntegerOverflow=on  InputSameDT=on
  CNTRIM : Product  InputSameDT=on  SaturateOnIntegerOverflow=on  OutDataTypeStr=Inherit: Same as first input
  CNWAF : Lookup2D  RowIndex=matnwaf(2:4,1)  ColumnIndex=matnwaf(1,2:4)  Table=matnwaf(2:4,2:4)  SaturateOnIntegerOverflow=on  InputSameDT=on
  CNWMH : Lookup2D  RowIndex=matnwmh(2:10,1)  ColumnIndex=matnwmh(1,2:10)  Table=matnwmh(2:10,2:10)  SaturateOnIntegerOverflow=on  InputSameDT=on
  Demux : Demux  Outputs=[1 1 1 1 1 1 1 1 1 1 1 1 1 1 1 1 1 1]
      settings: DisplayOption=none
  Neg : Gain  Gain=-1  SaturateOnIntegerOverflow=on  OutDataTypeStr=Inherit: Same as input  ParamDataTypeStr=Inherit: Same as input
  Sum : Sum  Inputs=+++  InputSameDT=on  SaturateOnIntegerOverflow=on  OutDataTypeStr=Inherit: Same as first input
  Sum1 : Sum  InputSameDT=on  SaturateOnIntegerOverflow=on  OutDataTypeStr=Inherit: Same as first input
  Sum2 : Sum  InputSameDT=on  SaturateOnIntegerOverflow=on  OutDataTypeStr=Inherit: Same as first input
  Terminator_{1..8} (8 alike) : Terminator
  zero : Constant  Value=0
  out_1 : Outport
  "out_2 " : Outport  Port=2
  wires:
  Demux/18 -> Terminator_8/1
  Demux/16 -> Terminator_7/1
  Demux/15 -> Terminator_6/1
  Demux/12 -> Terminator_5/1
  Demux/11 -> Terminator_4/1
  Demux/8 -> Terminator_3/1
  Demux/7 -> Terminator_2/1
  Demux/2 -> Terminator_1/1
  Sum/1 -> CNGUST/3, CNB/2
  CNR/1 -> CN/6
  CNB/1 -> CN/1
  CNDR/1 -> CN/3
  CNRTAM/1 -> CNTRIM/2
  CNRUAF/1 -> CNDR/2
  Sum1/1 -> CNDA/2
  Abs/1 -> CNBAB/1
  CN/1 -> out_1/1
  Demux/4 -> CNBAF/2, CNBAB/2, CNWAF/2, CNRTAM/2, CNPAF/2, CNRAF/2, CNRUAF/2
  Demux/5 -> CNB/1, Abs/1
  CNWAF/1 -> Sum1/1
  CNWMH/1 -> Sum1/2
  Demux/14 -> CNBAF/1, CNWAF/1, CNPAF/1, CNRAF/1, CNRUAF/1
  Demux/6 -> CNBMH/1, CNWMH/1, CNPMH/1
  CNBAF/1 -> Sum/1
  CNPAF/1 -> Sum2/1
  CNPMH/1 -> Sum2/2
  CNRAF/1 -> Neg/1, CNR/2
  Neg/1 -> CNGUST/7
  CNGUST/1 -> "out_2 "/1
  zero/1 -> CNGUST/2, CNGUST/4, CNGUST/5, CNGUST/6, CNGUST/1
  in_1/1 -> Demux/1
  Demux/17 -> CNBMH/2, CNRTAM/1, CNPMH/2, CNWMH/2
  CNDA/1 -> CN/2
  CNP/1 -> CN/5
  CNTRIM/1 -> CN/4
  Sum2/1 -> CNGUST/8, CNP/2
  Demux/13 -> CNTRIM/1
  Demux/10 -> CNDR/1
  Demux/9 -> CNDA/1
  Demux/1 -> CNP/1
  Demux/3 -> CNR/1
  CNBMH/1 -> Sum/2
  CNBAB/1 -> Sum/3

== system Citation/Cessna Citation 500/Citation model DASMAT/AIRCRAFT MODEL/AFM/Aeromod/SubSystem/model/CXGUST CZGUST ==
  CD : Inport
  CL : Inport  Port=2
  x : Inport  Port=3
  gust : Inport  Port=4
  CDalpha : Constant  Value=0.57
  CLalpha : Constant  Value=5.51
  CX/ ag : Sum  Inputs=+-  InputSameDT=on  SaturateOnIntegerOverflow=on  OutDataTypeStr=Inherit: Same as first input
  CX/ ug : Gain  Gain=2  SaturateOnIntegerOverflow=on  OutDataTypeStr=Inherit: Same as input  ParamDataTypeStr=Inherit: Same as input
  CXGUST : DotProduct  InputSameDT=on  OutDataTypeStr=Inherit: Inherit via internal rule
  CXbody : Fcn  Expr=-u[13]*cos(u[5])+u[14]*sin(u[5])
  CZ/ ag : Gain  Gain=-1  SaturateOnIntegerOverflow=on  OutDataTypeStr=Inherit: Same as input  ParamDataTypeStr=Inherit: Same as input
  CZ/ ug : Gain  Gain=2  SaturateOnIntegerOverflow=on  OutDataTypeStr=Inherit: Same as input  ParamDataTypeStr=Inherit: Same as input
  CZGUST : DotProduct  InputSameDT=on  OutDataTypeStr=Inherit: Inherit via internal rule
  CZbody : Fcn  Expr=-u[14]*cos(u[5])-u[13]*sin(u[5])
  Mux : Mux  Inputs=[12 1 1]
  Mux1 : Mux  Inputs=8
  Mux2 : Mux  Inputs=8
  zero : Constant  Value=0
  zero1 : Constant  Value=0
  "out_1 " : Outport
  "out_2 " : Outport  Port=2
  wires:
  zero1/1 -> Mux2/3, Mux2/7, Mux2/8, Mux2/6, Mux2/5, Mux2/4
  CZ/ ag/1 -> Mux2/2
  zero/1 -> Mux1/3, Mux1/7, Mux1/8, Mux1/6, Mux1/5, Mux1/4
  CX/ ag/1 -> Mux1/2
  CZGUST/1 -> "out_2 "/1
  CXGUST/1 -> "out_1 "/1
  gust/1 -> CZGUST/2, CXGUST/2
  Mux2/1 -> CZGUST/1
  Mux1/1 -> CXGUST/1
  Mux/1 -> CXbody/1, CZbody/1
  CL/1 -> CX/ ag/1, Mux/3
  CD/1 -> Mux/2
  x/1 -> Mux/1
  CDalpha/1 -> CX/ ag/2
  CLalpha/1 -> CZ/ ag/1
  CZbody/1 -> CZ/ ug/1
  CX/ ug/1 -> Mux1/1
  CXbody/1 -> CX/ ug/1
  CZ/ ug/1 -> Mux2/1

== system Citation/Cessna Citation 500/Citation model DASMAT/AIRCRAFT MODEL/AFM/Aeromod/SubSystem/model/CYCAL ==
  in_1 : Inport
  Abs : Abs  SaturateOnIntegerOverflow=on
  CY : Sum  Inputs=+++++  InputSameDT=on  SaturateOnIntegerOverflow=on  OutDataTypeStr=Inherit: Same as first input
  CY/ BETA : Sum  InputSameDT=on  SaturateOnIntegerOverflow=on  OutDataTypeStr=Inherit: Same as first input
  CYBAB : Lookup2D  RowIndex=matybab(2:5,1)  ColumnIndex=matybab(1,2:5)  Table=matybab(2:5,2:5)  SaturateOnIntegerOverflow=on  InputSameDT=on
  CYBAF : Lookup2D  RowIndex=matybaf(2:3,1)  ColumnIndex=matybaf(1,2:3)  Table=matybaf(2:3,2:3)  SaturateOnIntegerOverflow=on  InputSameDT=on
  CYBETA : Product  InputSameDT=on  SaturateOnIntegerOverflow=on  OutDataTypeStr=Inherit: Same as first input
  CYBUAF : Lookup2D  RowIndex=matbuaf(2:3,1)  ColumnIndex=matbuaf(1,2:3)  Table=matbuaf(2:3,2:3)  SaturateOnIntegerOverflow=on  InputSameDT=on
  CYBUC : Product  InputSameDT=on  SaturateOnIntegerOverflow=on  OutDataTypeStr=Inherit: Same as first input
  CYDA : Product  InputSameDT=on  SaturateOnIntegerOverflow=on  OutDataTypeStr=Inherit: Same as first input
  CYDR : Product  Inputs=3  InputSameDT=on  SaturateOnIntegerOverflow=on  OutDataTypeStr=Inherit: Same as first input
  CYGUST : Mux  Inputs=8
  CYR : Product  InputSameDT=on  SaturateOnIntegerOverflow=on  OutDataTypeStr=Inherit: Same as first input
  CYRAF : Lookup2D  RowIndex=matyraf(2:3,1)  ColumnIndex=matyraf(1,2:3)  Table=matyraf(2:3,2:3)  SaturateOnIntegerOverflow=on  InputSameDT=on
  CYRUAF : Lookup2D  RowIndex=matyuaf(2:3,1)  ColumnIndex=matyuaf(1,2:3)  Table=matyuaf(2:3,2:3)  SaturateOnIntegerOverflow=on  InputSameDT=on
  CYWAF : Lookup2D  RowIndex=matywaf(2:3,1)  ColumnIndex=matywaf(1,2:3)  Table=matywaf(2:3,2:3)  SaturateOnIntegerOverflow=on  InputSameDT=on
  Demux : Demux  Outputs=[1 1 1 1 1 1 1 1 1 1 1 1 1 1 1 1 1 1]
      settings: DisplayOption=none
  KUUT : Lookup  InputValues=matuut(1,:)  Table=matuut(2,:)  SaturateOnIntegerOverflow=on
  LSFACT : Subsystem
  Prod : Product  InputSameDT=on  SaturateOnIntegerOverflow=on  OutDataTypeStr=Inherit: Same as first input
  Sum : Sum  InputSameDT=on  SaturateOnIntegerOverflow=on  OutDataTypeStr=Inherit: Same as first input
  Terminator_{1..11} (11 alike) : Terminator
  zero : Constant  Value=0
  out_1 : Outport
  out_2 : Outport  Port=2
  wires:
  Demux/18 -> Terminator_11/1
  Demux/17 -> Terminator_10/1
  Demux/16 -> Terminator_9/1
  Demux/13 -> Terminator_8/1
  Demux/12 -> Terminator_7/1
  Demux/11 -> Terminator_6/1
  Demux/8 -> Terminator_5/1
  Demux/7 -> Terminator_4/1
  Demux/6 -> Terminator_3/1
  Demux/2 -> Terminator_2/1
  Demux/1 -> Terminator_1/1
  CY/ BETA/1 -> CYGUST/3
  CYBUAF/1 -> Prod/1
  CYBUC/1 -> CY/5
  CYR/1 -> CY/4
  CYBETA/1 -> CY/1
  CYRAF/1 -> CYR/2
  CYWAF/1 -> CYDA/2
  CYBAB/1 -> Sum/2
  CYBAF/1 -> Sum/1
  Abs/1 -> CYBAB/1
  CY/1 -> out_1/1
  KUUT/1 -> Prod/2
  Demux/14 -> CYBAF/1, CYRUAF/1, CYRAF/1, CYBUAF/1, CYWAF/1
  Demux/5 -> CYBETA/1, Abs/1, CYBUC/1
  Demux/4 -> CYBAF/2, CYWAF/2, CYRAF/2, CYBUAF/2, CYRUAF/2, CYBAB/2
  CYGUST/1 -> out_2/1
  zero/1 -> CYGUST/2, CYGUST/7, CYGUST/8, CYGUST/6, CYGUST/5, CYGUST/4, CYGUST/1
  in_1/1 -> Demux/1
  CYRUAF/1 -> CYDR/2
  Demux/10 -> CYDR/1, LSFACT/1(deltar)
  Sum/1 -> CY/ BETA/1, CYBETA/2
  Prod/1 -> CY/ BETA/2, CYBUC/2
  CYDA/1 -> CY/2
  CYDR/1 -> CY/3
  Demux/3 -> CYR/1
  Demux/15 -> KUUT/1
  Demux/9 -> CYDA/1
  LSFACT/1(LSFACT) -> CYDR/3

== system Citation/Cessna Citation 500/Citation model DASMAT/AIRCRAFT MODEL/EFM/Engmod/Citation eng_mod/Subsystem1/JT15 Dynamic ==
  In1 : Inport
  Demux : Demux  Outputs=32
      settings: DisplayOption=none
  Mux : Mux  Inputs=11
  Subsystem : Subsystem
  Out1 : Outport
  wires:
  Demux/32 -> Subsystem/32(Deng)
  Demux/31 -> Subsystem/31(VIAS)
  Demux/30 -> Subsystem/30(VCAS)
  Demux/29 -> Subsystem/29(VEAS)
  Demux/28 -> Subsystem/28(temptot)
  Demux/27 -> Subsystem/27(ptot)
  Demux/26 -> Subsystem/26(qrel)
  Demux/25 -> Subsystem/25(qc)
  Demux/24 -> Subsystem/24(Reynl)
  Demux/23 -> Subsystem/23(qdyn)
  Demux/22 -> Subsystem/22(Mach)
  Demux/21 -> Subsystem/21(Vsound)
  Demux/20 -> Subsystem/20(Hgeopot)
  Demux/19 -> Subsystem/19(hradio)
  Demux/18 -> Subsystem/18(hpress)
  Demux/17 -> Subsystem/17(grav)
  Demux/16 -> Subsystem/16(temp)
  Demux/15 -> Subsystem/15(rho)
  Demux/14 -> Subsystem/14(pstat)
  Demux/13 -> Subsystem/13(ut)
  Demux/12 -> Subsystem/12(ye)
  Demux/11 -> Subsystem/11(xe)
  Demux/10 -> Subsystem/10(he)
  Demux/9 -> Subsystem/9(psi)
  Demux/8 -> Subsystem/8(theta)
  Demux/7 -> Subsystem/7(phi)
  Demux/6 -> Subsystem/6(beta)
  Demux/5 -> Subsystem/5(alpha)
  Demux/4 -> Subsystem/4(VTAS)
  Demux/3 -> Subsystem/3(rbody)
  Demux/2 -> Subsystem/2(qbody)
  Demux/1 -> Subsystem/1(pbody)
  Subsystem/2(FF) -> Mux/2
  Subsystem/3(N1) -> Mux/3
  Subsystem/4(N2) -> Mux/4
  Subsystem/5(N1c) -> Mux/5
  Subsystem/6(N2c) -> Mux/6
  Subsystem/7(WT) -> Mux/7
  Subsystem/8(ITT) -> Mux/8
  Subsystem/9(EGT) -> Mux/9
  Subsystem/10(OILT) -> Mux/10
  Subsystem/11(OILP) -> Mux/11
  Subsystem/1(Tn) -> Mux/1
  In1/1 -> Demux/1
  Mux/1 -> Out1/1

== system Citation/Cessna Citation 500/Citation model DASMAT/AIRCRAFT MODEL/EFM/Engmod/Citation eng_mod/Subsystem1/JT15 Dynamic1 ==
  In1 : Inport
  Demux : Demux  Outputs=32
      settings: DisplayOption=none
  Mux : Mux  Inputs=11
  Subsystem : Subsystem
  Out1 : Outport
  wires:
  Demux/32 -> Subsystem/32(Deng)
  Demux/31 -> Subsystem/31(VIAS)
  Demux/30 -> Subsystem/30(VCAS)
  Demux/29 -> Subsystem/29(VEAS)
  Demux/28 -> Subsystem/28(temptot)
  Demux/27 -> Subsystem/27(ptot)
  Demux/26 -> Subsystem/26(qrel)
  Demux/25 -> Subsystem/25(qc)
  Demux/24 -> Subsystem/24(Reynl)
  Demux/23 -> Subsystem/23(qdyn)
  Demux/22 -> Subsystem/22(Mach)
  Demux/21 -> Subsystem/21(Vsound)
  Demux/20 -> Subsystem/20(Hgeopot)
  Demux/19 -> Subsystem/19(hradio)
  Demux/18 -> Subsystem/18(hpress)
  Demux/17 -> Subsystem/17(grav)
  Demux/16 -> Subsystem/16(temp)
  Demux/15 -> Subsystem/15(rho)
  Demux/14 -> Subsystem/14(pstat)
  Demux/13 -> Subsystem/13(ut)
  Demux/12 -> Subsystem/12(ye)
  Demux/11 -> Subsystem/11(xe)
  Demux/10 -> Subsystem/10(he)
  Demux/9 -> Subsystem/9(psi)
  Demux/8 -> Subsystem/8(theta)
  Demux/7 -> Subsystem/7(phi)
  Demux/6 -> Subsystem/6(beta)
  Demux/5 -> Subsystem/5(alpha)
  Demux/4 -> Subsystem/4(VTAS)
  Demux/3 -> Subsystem/3(rbody)
  Demux/2 -> Subsystem/2(qbody)
  Demux/1 -> Subsystem/1(pbody)
  Subsystem/2(FF) -> Mux/2
  Subsystem/3(N1) -> Mux/3
  Subsystem/4(N2) -> Mux/4
  Subsystem/5(N1c) -> Mux/5
  Subsystem/6(N2c) -> Mux/6
  Subsystem/7(WT) -> Mux/7
  Subsystem/8(ITT) -> Mux/8
  Subsystem/9(EGT) -> Mux/9
  Subsystem/10(OILT) -> Mux/10
  Subsystem/11(OILP) -> Mux/11
  Subsystem/1(Tn) -> Mux/1
  In1/1 -> Demux/1
  Mux/1 -> Out1/1

== system Citation/Cessna Citation 500/Citation model DASMAT/AIRCRAFT MODEL/AFM/Aeromod/SubSystem/model/CDCAL/KBASD ==
  hcg : Inport
  deltaf : Inport  Port=2
  VEAS : Inport  Port=3
  Constant : Constant
  Fcn : Fcn  Expr=0.2-u[1]
  Fcn1 : Fcn  Expr=u[2]*(u[1]*180/pi-15)*0.04*(100-u[3])/30
  Fcn2 : Fcn  Expr=1-0.6*u[1]
  KGEDHR : Lookup  InputValues=matedhr(1,:)  Table=matedhr(2,:)  SaturateOnIntegerOverflow=on
  Mux : Mux  Inputs=3
  Sat : Saturate  UpperLimit=1  LowerLimit=0
  Switch : Switch  SaturateOnIntegerOverflow=on  InputSameDT=on
  KBASD : Outport
  wires:
  KGEDHR/1 -> Mux/2
  deltaf/1 -> Mux/1, Fcn/1
  Fcn/1 -> Switch/2
  Constant/1 -> Switch/1
  Switch/1 -> KBASD/1
  VEAS/1 -> Mux/3
  hcg/1 -> KGEDHR/1
  Mux/1 -> Fcn1/1
  Sat/1 -> Fcn2/1
  Fcn1/1 -> Sat/1
  Fcn2/1 -> Switch/3

== system Citation/Cessna Citation 500/Citation model DASMAT/AIRCRAFT MODEL/AFM/Aeromod/SubSystem/model/CLCAL/CLGEAF ==
  alpha : Inport
  deltaf : Inport  Port=2
  Prod : Product  InputSameDT=on  SaturateOnIntegerOverflow=on  OutDataTypeStr=Inherit: Same as first input
  Sat : Saturate  UpperLimit=0.04  LowerLimit=-inf
  Sum : Sum  InputSameDT=on  SaturateOnIntegerOverflow=on  OutDataTypeStr=Inherit: Same as first input
  VDOMMYR37 : Lookup  InputValues=vdommyr37(1,:)  Table=vdommyr37(2,:)  SaturateOnIntegerOverflow=on
  VDOMMYR40 : Gain  Gain=1.6  SaturateOnIntegerOverflow=on  OutDataTypeStr=Inherit: Same as input  ParamDataTypeStr=Inherit: Same as input
  rad2deg : Gain  Gain=(180/pi)  SaturateOnIntegerOverflow=on  OutDataTypeStr=Inherit: Same as input  ParamDataTypeStr=Inherit: Same as input
  CLGEAF : Outport
  wires:
  VDOMMYR37/1 -> VDOMMYR40/1, Prod/2
  rad2deg/1 -> Prod/1
  Sat/1 -> rad2deg/1
  alpha/1 -> Sat/1
  deltaf/1 -> VDOMMYR37/1
  VDOMMYR40/1 -> Sum/2
  Prod/1 -> Sum/1
  Sum/1 -> CLGEAF/1

== system Citation/Cessna Citation 500/Citation model DASMAT/AIRCRAFT MODEL/AFM/Aeromod/SubSystem/model/CLCAL/SP0 ==
  deltae : Inport
  Abs : Abs  SaturateOnIntegerOverflow=on
  Fcn : Fcn  Expr=(0.087+0.25*(u[1]-0.087))/(u[1]+1e-11)
  Prod : Product  InputSameDT=on  SaturateOnIntegerOverflow=on  OutDataTypeStr=Inherit: Same as first input
  Sat : Saturate  UpperLimit=1  LowerLimit=-inf
  SP0 : Outport
  wires:
  deltae/1 -> Prod/1, Abs/1
  Sat/1 -> Prod/2
  Fcn/1 -> Sat/1
  Abs/1 -> Fcn/1
  Prod/1 -> SP0/1

== system Citation/Cessna Citation 500/Citation model DASMAT/AIRCRAFT MODEL/AFM/Aeromod/SubSystem/model/CLLCAL/CIBAB ==
  note: 02-11-2000
      | Modified by A. R. Veldhuijzen
      | sftable3.m was replaced with table3.dll
      | X and Y are exchanged in this Mathworks implementation
  x0 : Inport
  y0 : Inport  Port=2
  z0 : Inport  Port=3
  Mux : Mux  Inputs=3
  S-function : S-Function  FunctionName=table3  Parameters=yindex, xindex ,zindex, table  SFunctionDeploymentMode=off  EnableBusSupport=off
  out_1 : Outport
  wires:
  z0/1 -> Mux/3
  y0/1 -> Mux/1
  x0/1 -> Mux/2
  Mux/1 -> S-function/1
  S-function/1 -> out_1/1

== system Citation/Cessna Citation 500/Citation model DASMAT/AIRCRAFT MODEL/AFM/Aeromod/SubSystem/model/CLLCAL/LFACT ==
  hcg : Inport
  Sat : Saturate  UpperLimit=1  LowerLimit=0
  hrunway : Fcn  Expr=1-(u[1]-1)/30
  LFACT : Outport
  wires:
  Sat/1 -> LFACT/1
  hcg/1 -> hrunway/1
  hrunway/1 -> Sat/1

== system Citation/Cessna Citation 500/Citation model DASMAT/AIRCRAFT MODEL/AFM/Aeromod/SubSystem/model/CMCAL/EALPHA ==
  alpha : Inport
  deltaf : Inport  Port=2
  Fcn : Fcn  Expr=1-u[1]*u[2]
  Mux : Mux  Inputs=2
  Sat : Saturate  UpperLimit=1  LowerLimit=0
  Sum : Sum  Inputs=+-  InputSameDT=on  SaturateOnIntegerOverflow=on  OutDataTypeStr=Inherit: Same as first input
  ealphag : Lookup  InputValues=ealphag(1,:)  Table=ealphag(2,:)  SaturateOnIntegerOverflow=on
  ealphas : Lookup  InputValues=ealphas(1,:)  Table=ealphas(2,:)  SaturateOnIntegerOverflow=on
  EALPHA : Outport
  wires:
  deltaf/1 -> ealphag/1, ealphas/1
  alpha/1 -> Sum/1
  Mux/1 -> Fcn/1
  ealphag/1 -> Mux/2
  ealphas/1 -> Sum/2
  Sum/1 -> Mux/1
  Fcn/1 -> Sat/1
  Sat/1 -> EALPHA/1

== system Citation/Cessna Citation 500/Citation model DASMAT/AIRCRAFT MODEL/AFM/Aeromod/SubSystem/model/CMCAL/LFCMEGAF ==
  alpha : Inport
  Abs : Abs  SaturateOnIntegerOverflow=on
  Fcn : Fcn  Expr=1-5*u[1]
  Neg : Gain  Gain=-1  SaturateOnIntegerOverflow=on  OutDataTypeStr=Inherit: Same as input  ParamDataTypeStr=Inherit: Same as input
  Sat : Saturate  UpperLimit=inf  LowerLimit=0.25
  LFCMEGAF : Outport
  wires:
  Fcn/1 -> Sat/1
  alpha/1 -> Abs/1
  Abs/1 -> Fcn/1
  Sat/1 -> Neg/1
  Neg/1 -> LFCMEGAF/1

== system Citation/Cessna Citation 500/Citation model DASMAT/AIRCRAFT MODEL/AFM/Aeromod/SubSystem/model/CYCAL/LSFACT ==
  deltar : Inport
  Abs : Abs  SaturateOnIntegerOverflow=on
  Fcn : Fcn  Expr=0.06981/u[1]+2*(u[1]-0.06981)
  Sat : Saturate  UpperLimit=inf  LowerLimit=0.06981
  LSFACT : Outport
  wires:
  deltar/1 -> Abs/1
  Abs/1 -> Sat/1
  Sat/1 -> Fcn/1
  Fcn/1 -> LSFACT/1

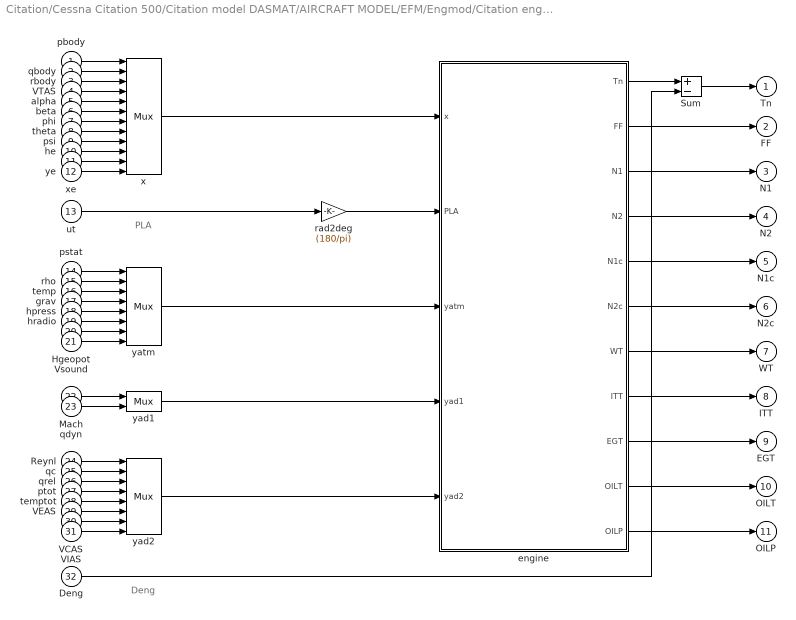
== system Citation/Cessna Citation 500/Citation model DASMAT/AIRCRAFT MODEL/EFM/Engmod/Citation eng_mod/Subsystem1/JT15 Dynamic/Subsystem ==
  note: Deng
  note: PLA
  pbody : Inport
  qbody : Inport  Port=2
  rbody : Inport  Port=3
  VTAS : Inport  Port=4
  alpha : Inport  Port=5
  beta : Inport  Port=6
  phi : Inport  Port=7
  theta : Inport  Port=8
  psi : Inport  Port=9
  he : Inport  Port=10
  xe : Inport  Port=11
  ye : Inport  Port=12
  ut : Inport  Port=13
  pstat : Inport  Port=14
  rho : Inport  Port=15
  temp : Inport  Port=16
  grav : Inport  Port=17
  hpress : Inport  Port=18
  hradio : Inport  Port=19
  Hgeopot : Inport  Port=20
  Vsound : Inport  Port=21
  Mach : Inport  Port=22
  qdyn : Inport  Port=23
  Reynl : Inport  Port=24
  qc : Inport  Port=25
  qrel : Inport  Port=26
  ptot : Inport  Port=27
  temptot : Inport  Port=28
  VEAS : Inport  Port=29
  VCAS : Inport  Port=30
  VIAS : Inport  Port=31
  Deng : Inport  Port=32
  Sum : Sum  Inputs=+-  InputSameDT=on  SaturateOnIntegerOverflow=on  OutDataTypeStr=Inherit: Same as first input
  engine : Subsystem
  rad2deg : Gain  Gain=(180/pi)  SaturateOnIntegerOverflow=on  OutDataTypeStr=Inherit: Same as input  ParamDataTypeStr=Inherit: Same as input
  x : Mux  Inputs=12
  yad1 : Mux  Inputs=2
  yad2 : Mux  Inputs=8
  yatm : Mux  Inputs=8
  Tn : Outport
  FF : Outport  Port=2
  N1 : Outport  Port=3
  N2 : Outport  Port=4
  N1c : Outport  Port=5
  N2c : Outport  Port=6
  WT : Outport  Port=7
  ITT : Outport  Port=8
  EGT : Outport  Port=9
  OILT : Outport  Port=10
  OILP : Outport  Port=11
  wires:
  Deng/1 -> Sum/2
  engine/1(Tn) -> Sum/1
  Sum/1 -> Tn/1
  Vsound/1 -> yatm/8
  engine/11(OILP) -> OILP/1
  engine/10(OILT) -> OILT/1
  rad2deg/1 -> engine/2(PLA)
  ut/1 -> rad2deg/1
  engine/9(EGT) -> EGT/1
  engine/8(ITT) -> ITT/1
  engine/7(WT) -> WT/1
  engine/6(N2c) -> N2c/1
  engine/5(N1c) -> N1c/1
  engine/4(N2) -> N2/1
  engine/3(N1) -> N1/1
  engine/2(FF) -> FF/1
  yad1/1 -> engine/4(yad1)
  yatm/1 -> engine/3(yatm)
  yad2/1 -> engine/5(yad2)
  qdyn/1 -> yad1/2
  Mach/1 -> yad1/1
  Reynl/1 -> yad2/1
  qc/1 -> yad2/2
  VCAS/1 -> yad2/7
  temptot/1 -> yad2/5
  qrel/1 -> yad2/3
  VIAS/1 -> yad2/8
  VEAS/1 -> yad2/6
  ptot/1 -> yad2/4
  ye/1 -> x/12
  xe/1 -> x/11
  he/1 -> x/10
  psi/1 -> x/9
  VTAS/1 -> x/4
  beta/1 -> x/6
  theta/1 -> x/8
  rbody/1 -> x/3
  alpha/1 -> x/5
  phi/1 -> x/7
  qbody/1 -> x/2
  pbody/1 -> x/1
  pstat/1 -> yatm/1
  rho/1 -> yatm/2
  Hgeopot/1 -> yatm/7
  hpress/1 -> yatm/5
  temp/1 -> yatm/3
  hradio/1 -> yatm/6
  grav/1 -> yatm/4
  x/1 -> engine/1(x)

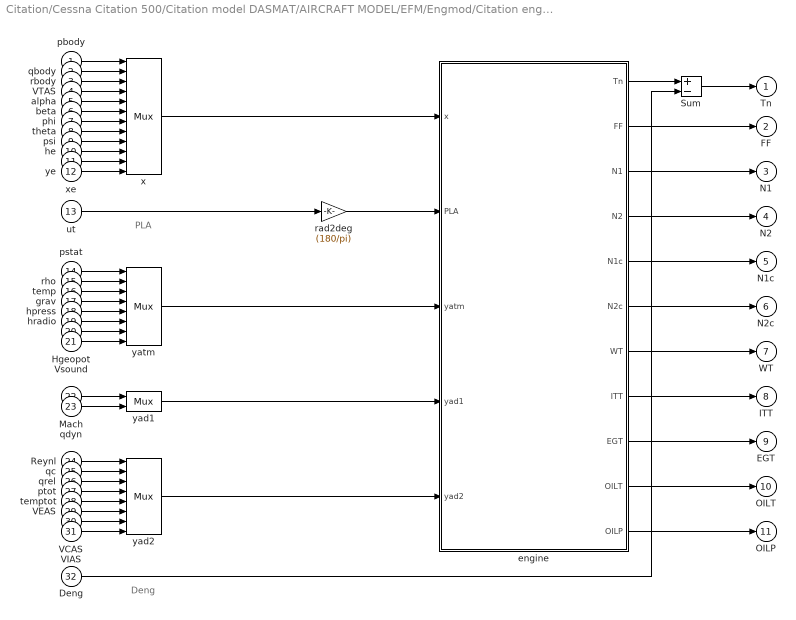
== system Citation/Cessna Citation 500/Citation model DASMAT/AIRCRAFT MODEL/EFM/Engmod/Citation eng_mod/Subsystem1/JT15 Dynamic1/Subsystem ==
  note: Deng
  note: PLA
  pbody : Inport
  qbody : Inport  Port=2
  rbody : Inport  Port=3
  VTAS : Inport  Port=4
  alpha : Inport  Port=5
  beta : Inport  Port=6
  phi : Inport  Port=7
  theta : Inport  Port=8
  psi : Inport  Port=9
  he : Inport  Port=10
  xe : Inport  Port=11
  ye : Inport  Port=12
  ut : Inport  Port=13
  pstat : Inport  Port=14
  rho : Inport  Port=15
  temp : Inport  Port=16
  grav : Inport  Port=17
  hpress : Inport  Port=18
  hradio : Inport  Port=19
  Hgeopot : Inport  Port=20
  Vsound : Inport  Port=21
  Mach : Inport  Port=22
  qdyn : Inport  Port=23
  Reynl : Inport  Port=24
  qc : Inport  Port=25
  qrel : Inport  Port=26
  ptot : Inport  Port=27
  temptot : Inport  Port=28
  VEAS : Inport  Port=29
  VCAS : Inport  Port=30
  VIAS : Inport  Port=31
  Deng : Inport  Port=32
  Sum : Sum  Inputs=+-  InputSameDT=on  SaturateOnIntegerOverflow=on  OutDataTypeStr=Inherit: Same as first input
  engine : Subsystem
  rad2deg : Gain  Gain=(180/pi)  SaturateOnIntegerOverflow=on  OutDataTypeStr=Inherit: Same as input  ParamDataTypeStr=Inherit: Same as input
  x : Mux  Inputs=12
  yad1 : Mux  Inputs=2
  yad2 : Mux  Inputs=8
  yatm : Mux  Inputs=8
  Tn : Outport
  FF : Outport  Port=2
  N1 : Outport  Port=3
  N2 : Outport  Port=4
  N1c : Outport  Port=5
  N2c : Outport  Port=6
  WT : Outport  Port=7
  ITT : Outport  Port=8
  EGT : Outport  Port=9
  OILT : Outport  Port=10
  OILP : Outport  Port=11
  wires:
  Deng/1 -> Sum/2
  engine/1(Tn) -> Sum/1
  Sum/1 -> Tn/1
  Vsound/1 -> yatm/8
  engine/11(OILP) -> OILP/1
  engine/10(OILT) -> OILT/1
  rad2deg/1 -> engine/2(PLA)
  ut/1 -> rad2deg/1
  engine/9(EGT) -> EGT/1
  engine/8(ITT) -> ITT/1
  engine/7(WT) -> WT/1
  engine/6(N2c) -> N2c/1
  engine/5(N1c) -> N1c/1
  engine/4(N2) -> N2/1
  engine/3(N1) -> N1/1
  engine/2(FF) -> FF/1
  yad1/1 -> engine/4(yad1)
  yatm/1 -> engine/3(yatm)
  yad2/1 -> engine/5(yad2)
  qdyn/1 -> yad1/2
  Mach/1 -> yad1/1
  Reynl/1 -> yad2/1
  qc/1 -> yad2/2
  VCAS/1 -> yad2/7
  temptot/1 -> yad2/5
  qrel/1 -> yad2/3
  VIAS/1 -> yad2/8
  VEAS/1 -> yad2/6
  ptot/1 -> yad2/4
  ye/1 -> x/12
  xe/1 -> x/11
  he/1 -> x/10
  psi/1 -> x/9
  VTAS/1 -> x/4
  beta/1 -> x/6
  theta/1 -> x/8
  rbody/1 -> x/3
  alpha/1 -> x/5
  phi/1 -> x/7
  qbody/1 -> x/2
  pbody/1 -> x/1
  pstat/1 -> yatm/1
  rho/1 -> yatm/2
  Hgeopot/1 -> yatm/7
  hpress/1 -> yatm/5
  temp/1 -> yatm/3
  hradio/1 -> yatm/6
  grav/1 -> yatm/4
  x/1 -> engine/1(x)
